simulink model "sampleModel1966"  (R2023a)
settings: Solver=VariableStepAuto  StartTime=0.0  StopTime=10.0  RelTol=1e-3
libraries: hdlsllib x3
settings Model: Creator=user1  LastModifiedBy=user1

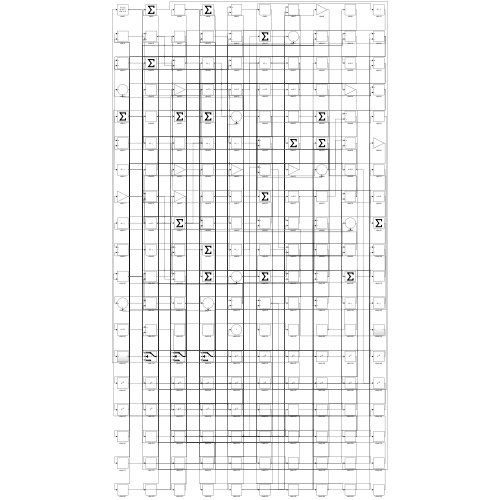
[thumbnail: Simulink's stored preview of the top-level diagram]
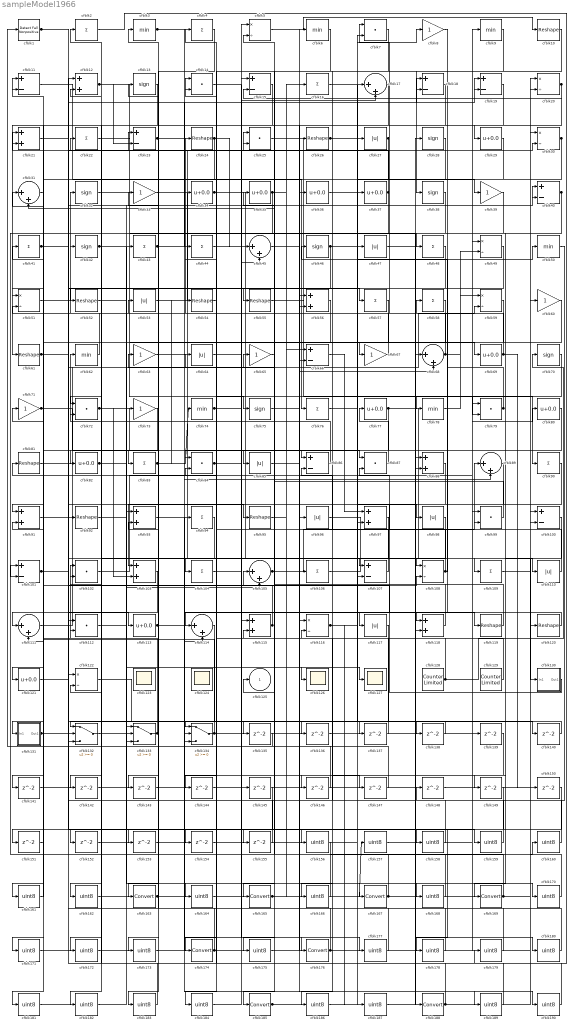
== system sampleModel1966 ==
  cfblk1 : hdlsllib/Logic and Bit Operations/Detect Fall Nonpositive  vinit=0  OutDataTypeStr=boolean
  cfblk{10,24,26,52,54..55,61,81,92,95,119..120} (12 alike) : Reshape
  cfblk{11,15,18..19,23,40,66,86,100..101,107} (11 alike) : Sum  Inputs=+-
  cfblk{7,14,25,72,79,84,87,99,102,112} (10 alike) : DotProduct  OutDataTypeStr=Inherit: Inherit via internal rule
  cfblk{12,21,56,88,91,93,97,103,115,118} (10 alike) : Sum
  cfblk{2,4,16,22,41,43..44,48,57..58,76,83,90,94,104,106,109} (17 alike) : Sum  Inputs=+
  cfblk{17,31,45,68,89,105,111,114} (8 alike) : Sum  Inputs=|++
  cfblk{5,20,30,49,51,59,108,116,122} (9 alike) : Product  Inputs=*/  RndMeth=Zero  SaturateOnIntegerOverflow=on
  cfblk{27,47,53,64,85,96,98,110,117} (9 alike) : Abs  SaturateOnIntegerOverflow=off
  cfblk{29,34..37,69,77,80,82,113,121} (11 alike) : Bias  Bias=0.0  SaturateOnIntegerOverflow=off
  cfblk{123..124,126..127} (4 alike) : Scope
      cfblk123 settings: Floating=on
      cfblk124 settings: Floating=on
  cfblk128 : hdlsllib/Sources/Counter Limited  uplimit=7  tsamp=-1
  cfblk129 : hdlsllib/Sources/Counter Limited  uplimit=7  tsamp=-1
  cfblk{13,28,32,38,42,46,70,75} (8 alike) : Signum
  cfblk130 : Subsystem
      settings: LibrarySourceBlock=|
      | hdlsllib/Ports &
      | Subsystems/Subsystem
  cfblk131 : Subsystem
      settings: LibrarySourceBlock=|
      | hdlsllib/Ports &
      | Subsystems/Subsystem
  cfblk132 : Switch  SaturateOnIntegerOverflow=off  InputSameDT=off
  cfblk133 : Switch  SaturateOnIntegerOverflow=off  InputSameDT=off
  cfblk134 : Switch  SaturateOnIntegerOverflow=off  InputSameDT=off
  cfblk{135..155} (21 alike) : Delay  SampleTime=1
  cfblk{156..162,164,166,168,170..173,175,177..184,186..187,189..190} (27 alike) : DataTypeConversion  OutDataTypeStr=uint8  SaturateOnIntegerOverflow=off  RndMeth=Floor
  cfblk{163,165,167,169,174,176,185,188} (8 alike) : DataTypeConversion  SaturateOnIntegerOverflow=off  RndMeth=Floor
  cfblk{3,6,9,50,62,74,78} (7 alike) : MinMax
  cfblk{8,33,39,60,63,65,67,71,73} (9 alike) : Gain
  cfblk125 : Outport  VectorParamsAs1DForOutWhenUnconnected=off
  wires:
  cfblk34/1 -> cfblk110/1, cfblk19/1
  cfblk95/1 -> cfblk16/1
  cfblk30/1 -> cfblk153/1, cfblk166/1
  cfblk78/1 -> cfblk59/1
  cfblk38/1 -> cfblk48/1
  cfblk12/1 -> cfblk75/1, cfblk23/2
  cfblk81/1 -> cfblk85/1
  cfblk33/1 -> cfblk108/1
  cfblk86/1 -> cfblk62/1
  cfblk9/1 -> cfblk38/1
  cfblk83/1 -> cfblk74/1, cfblk54/1, cfblk155/1
  cfblk66/1 -> cfblk97/1
  cfblk13/1 -> cfblk61/1
  cfblk117/1 -> cfblk132/1
  cfblk128/1 -> cfblk70/1, cfblk21/1
  cfblk70/1 -> cfblk84/1
  cfblk69/1 -> cfblk32/1, cfblk150/1
  cfblk11/1 -> cfblk76/1
  cfblk42/1 -> cfblk34/1, cfblk152/1, cfblk170/1
  cfblk68/1 -> cfblk24/1, cfblk7/1, cfblk49/2
  cfblk6/1 -> cfblk174/1
  cfblk55/1 -> cfblk90/1
  cfblk105/1 -> cfblk89/1, cfblk190/1
  cfblk111/1 -> cfblk59/2
  cfblk20/1 -> cfblk15/2, cfblk132/3, cfblk66/2
  cfblk25/1 -> cfblk69/1
  cfblk64/1 -> cfblk87/1
  cfblk130/1(Out1) -> cfblk105/1
  cfblk120/1 -> cfblk114/1
  cfblk5/1 -> cfblk10/1
  cfblk23/1 -> cfblk3/1, cfblk189/1
  cfblk77/1 -> cfblk130/1(In1), cfblk97/2
  cfblk133/1 -> cfblk102/1, cfblk91/2
  cfblk71/1 -> cfblk83/1, cfblk18/2
  cfblk101/1 -> cfblk25/1, cfblk108/2, cfblk19/2, cfblk151/1
  cfblk10/1 -> cfblk55/1
  cfblk15/1 -> cfblk131/1(In1)
  cfblk27/1 -> cfblk134/3, cfblk135/1
  cfblk16/1 -> cfblk39/1
  cfblk67/1 -> cfblk35/1
  cfblk79/1 -> cfblk46/1, cfblk53/1
  cfblk44/1 -> cfblk167/1
  cfblk53/1 -> cfblk5/1
  cfblk104/1 -> cfblk17/2
  cfblk107/1 -> cfblk4/1
  cfblk134/1 -> cfblk31/1, cfblk49/1, cfblk177/1
  cfblk88/1 -> cfblk185/1
  cfblk7/1 -> cfblk86/1
  cfblk131/1(Out1) -> cfblk64/1, cfblk41/1
  cfblk35/1 -> cfblk26/1, cfblk144/1
  cfblk93/1 -> cfblk176/1
  cfblk119/1 -> cfblk63/1
  cfblk1/1 -> cfblk57/1, cfblk159/1
  cfblk31/1 -> cfblk111/1
  cfblk115/1 -> cfblk22/1, cfblk21/2
  cfblk89/1 -> cfblk117/1
  cfblk24/1 -> cfblk111/2, cfblk45/1
  cfblk113/1 -> cfblk119/1, cfblk146/1
  cfblk100/1 -> cfblk169/1
  cfblk22/1 -> cfblk67/1
  cfblk92/1 -> cfblk43/1
  cfblk40/1 -> cfblk118/1, cfblk149/1
  cfblk87/1 -> cfblk77/1
  cfblk129/1 -> cfblk81/1
  cfblk37/1 -> cfblk23/1, cfblk101/2
  cfblk122/1 -> cfblk188/1
  cfblk18/1 -> cfblk51/1
  cfblk61/1 -> cfblk95/1, cfblk40/1
  cfblk57/1 -> cfblk91/1
  cfblk102/1 -> cfblk80/1
  cfblk51/1 -> cfblk42/1
  cfblk110/1 -> cfblk87/2
  cfblk76/1 -> cfblk50/1
  cfblk85/1 -> cfblk56/1
  cfblk72/1 -> cfblk115/1, cfblk103/2
  cfblk118/1 -> cfblk31/2
  cfblk39/1 -> cfblk72/1
  cfblk3/1 -> cfblk89/2, cfblk109/1
  cfblk21/1 -> cfblk113/1
  cfblk75/1 -> cfblk68/2
  cfblk103/1 -> cfblk121/1
  cfblk109/1 -> cfblk20/2
  cfblk74/1 -> cfblk30/2, cfblk126/1
  cfblk84/1 -> cfblk14/1, cfblk147/1
  cfblk43/1 -> cfblk114/2, cfblk18/1
  cfblk90/1 -> cfblk103/1
  cfblk106/1 -> cfblk9/1
  cfblk65/1 -> cfblk165/1
  cfblk14/1 -> cfblk107/1
  cfblk41/1 -> cfblk92/1, cfblk25/2
  cfblk46/1 -> cfblk56/2, cfblk140/1, cfblk162/1
  cfblk19/1 -> cfblk29/1
  cfblk36/1 -> cfblk79/2
  cfblk99/1 -> cfblk5/2
  cfblk49/1 -> cfblk132/2
  cfblk91/1 -> cfblk107/2
  cfblk28/1 -> cfblk163/1
  cfblk62/1 -> cfblk11/1
  cfblk26/1 -> cfblk98/1, cfblk8/1
  cfblk108/1 -> cfblk58/1, cfblk86/2
  cfblk8/1 -> cfblk78/1
  cfblk80/1 -> cfblk104/1
  cfblk82/1 -> cfblk127/1, cfblk105/2
  cfblk58/1 -> cfblk82/1
  cfblk32/1 -> cfblk118/2
  cfblk96/1 -> cfblk99/2
  cfblk17/1 -> cfblk52/1
  cfblk116/1 -> cfblk40/2, cfblk187/1
  cfblk45/1 -> cfblk106/1
  cfblk135/1 -> cfblk1/1
  cfblk59/1 -> cfblk136/1
  cfblk132/1 -> cfblk137/1
  cfblk137/1 -> cfblk116/1
  cfblk121/1 -> cfblk138/1
  cfblk138/1 -> cfblk134/1
  cfblk140/1 -> cfblk133/2
  cfblk56/1 -> cfblk141/1
  cfblk141/1 -> cfblk68/1
  cfblk114/1 -> cfblk142/1
  cfblk142/1 -> cfblk15/1
  cfblk4/1 -> cfblk143/1
  cfblk143/1 -> cfblk79/1
  cfblk144/1 -> cfblk20/1
  cfblk146/1 -> cfblk133/1
  cfblk147/1 -> cfblk115/2
  cfblk50/1 -> cfblk148/1
  cfblk148/1 -> cfblk30/1
  cfblk151/1 -> cfblk51/2
  cfblk152/1 -> cfblk134/2
  cfblk153/1 -> cfblk45/2
  cfblk54/1 -> cfblk154/1
  cfblk154/1 -> cfblk17/1
  cfblk155/1 -> cfblk12/2
  cfblk139/1 -> cfblk156/1
  cfblk157/1 -> cfblk139/1
  cfblk112/1 -> cfblk158/1
  cfblk158/1 -> cfblk116/2
  cfblk159/1 -> cfblk112/1
  cfblk156/1 -> cfblk160/1
  cfblk160/1 -> cfblk112/2
  cfblk60/1 -> cfblk161/1
  cfblk161/1 -> cfblk71/1
  cfblk162/1 -> cfblk60/1
  cfblk163/1 -> cfblk157/1, cfblk36/1
  cfblk52/1 -> cfblk164/1
  cfblk164/1 -> cfblk28/1
  cfblk165/1 -> cfblk7/2, cfblk66/1, cfblk37/1
  cfblk166/1 -> cfblk65/1
  cfblk167/1 -> cfblk11/2, cfblk84/2
  cfblk63/1 -> cfblk168/1
  cfblk168/1 -> cfblk44/1
  cfblk169/1 -> cfblk101/1, cfblk125/1
  cfblk170/1 -> cfblk100/1
  cfblk150/1 -> cfblk171/1
  cfblk171/1 -> cfblk100/2
  cfblk94/1 -> cfblk172/1
  cfblk172/1 -> cfblk96/1
  cfblk29/1 -> cfblk173/1
  cfblk173/1 -> cfblk94/1
  cfblk174/1 -> cfblk33/1, cfblk13/1
  cfblk97/1 -> cfblk175/1
  cfblk175/1 -> cfblk6/1
  cfblk176/1 -> cfblk12/1, cfblk99/1
  cfblk177/1 -> cfblk93/1
  cfblk149/1 -> cfblk178/1
  cfblk178/1 -> cfblk93/2
  cfblk2/1 -> cfblk179/1
  cfblk179/1 -> cfblk72/2
  cfblk47/1 -> cfblk180/1
  cfblk180/1 -> cfblk2/1
  cfblk73/1 -> cfblk181/1
  cfblk181/1 -> cfblk133/3
  cfblk48/1 -> cfblk182/1
  cfblk182/1 -> cfblk73/1
  cfblk145/1 -> cfblk183/1
  cfblk183/1 -> cfblk102/2
  cfblk98/1 -> cfblk184/1
  cfblk184/1 -> cfblk145/1
  cfblk185/1 -> cfblk47/1, cfblk27/1
  cfblk136/1 -> cfblk186/1
  cfblk186/1 -> cfblk88/1
  cfblk187/1 -> cfblk88/2
  cfblk188/1 -> cfblk14/2, cfblk120/1
  cfblk189/1 -> cfblk122/1
  cfblk190/1 -> cfblk122/2

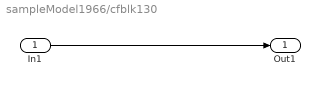
== system sampleModel1966/cfblk130 ==
  In1 : Inport
  Out1 : Outport
  wires:
  In1/1 -> Out1/1

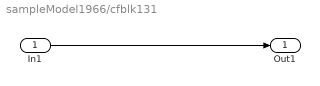
== system sampleModel1966/cfblk131 ==
  In1 : Inport
  Out1 : Outport
  wires:
  In1/1 -> Out1/1
